simulink model "Audio_Transmission_1_"  (R2025a)
settings: Solver=VariableStepAuto  StartTime=0.0  StopTime=8  RelTol=1e-3
libraries: commanapbnd3 x6, commchan3 x3, dspsnks4 x1, dspvision x1
settings Model: Creator=sriva  LastModifiedBy=sriva

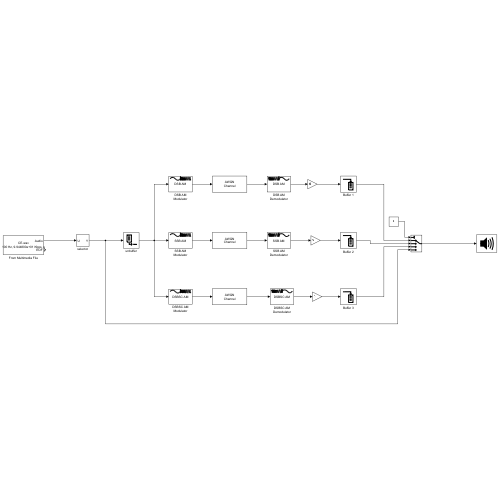
[thumbnail: Simulink's stored preview of the top-level diagram]
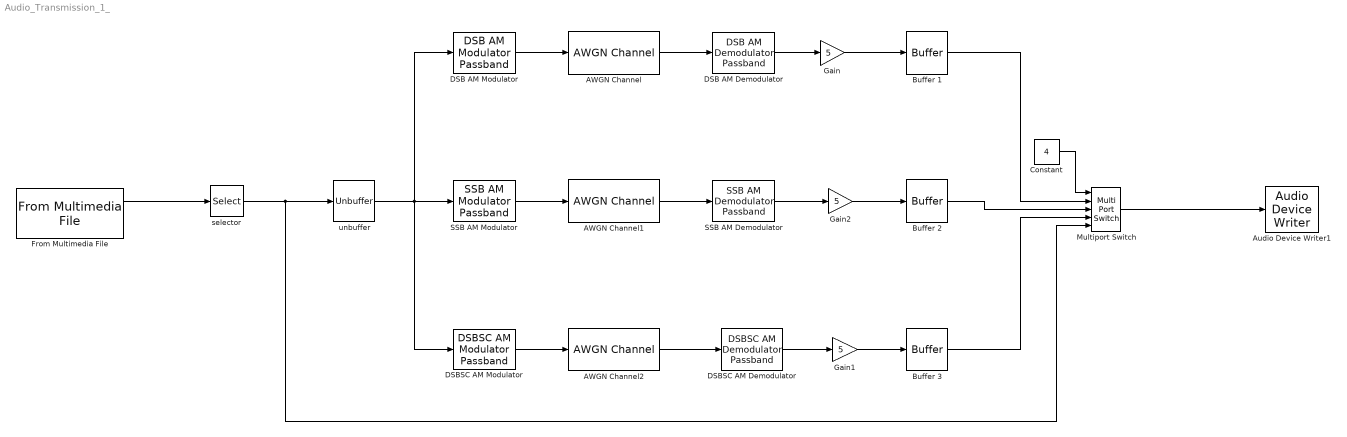
== system Audio_Transmission_1_ ==
  AWGN Channel : commchan3/AWGN Channel  LegacyMode=off  NoiseMethod="Signal to noise ratio  (SNR)"  noiseMode="Signal to noise ratio  (SNR)"  EbNo=10  EsNo=10  SNR=30  BitsPerSymbol=1  SignalPower=1  SpecifySymbolPeriod=off  SamplesPerSymbol=1  SymbolPeriod=1  VarianceSource=Parameter  Variance=1  RandomStream=Global stream  Seed=67  SimulateUsing=Code generation
  AWGN Channel1 : commchan3/AWGN Channel  LegacyMode=off  NoiseMethod="Signal to noise ratio  (SNR)"  noiseMode="Signal to noise ratio  (SNR)"  EbNo=10  EsNo=10  SNR=30  BitsPerSymbol=1  SignalPower=1  SpecifySymbolPeriod=off  SamplesPerSymbol=1  SymbolPeriod=1  VarianceSource=Parameter  Variance=1  RandomStream=Global stream  Seed=67  SimulateUsing=Code generation
  AWGN Channel2 : commchan3/AWGN Channel  LegacyMode=off  NoiseMethod="Signal to noise ratio  (SNR)"  noiseMode="Signal to noise ratio  (SNR)"  EbNo=10  EsNo=10  SNR=1000  BitsPerSymbol=1  SignalPower=1  SpecifySymbolPeriod=off  SamplesPerSymbol=1  SymbolPeriod=1  VarianceSource=Parameter  Variance=1  RandomStream=Global stream  Seed=67  SimulateUsing=Code generation
  Audio Device Writer1 : dspsnks4/Audio Device Writer  Driver=DirectSound  Device=Default  InheritSampleRate=on  SampleRate=1024  BitDepth=16-bit integer  BufferSize=4096  NumBuffers=10  DefaultOutputChannelMapping=on  OutputChannelMapping=1:2  OutputNumUnderrunSamples=off  DriverIdx=1  DeviceWarnFlag=''
  Buffer 1 : Buffer  N=1024  OutputFrames=off
  Buffer 2 : Buffer  N=1024  OutputFrames=off
  Buffer 3 : Buffer  N=1024  OutputFrames=off
  Constant : Constant  Value=4
  "DSB AM Demodulator " : commanapbnd3/DSB AM Demodulator Passband  Fc=10000  Ph=0  method=Butterworth  n=6  cf=5000  Rp=0.1  Rs=50  Offset=1
  "DSB AM Modulator " : commanapbnd3/DSB AM Modulator Passband  Fc=10000  Ph=0  Offset=1
  DSBSC AM Demodulator : commanapbnd3/DSBSC AM Demodulator Passband  Fc=10000  Ph=0  method=Butterworth  n=6  cf=5000  Rp=0.1  Rs=50
  "DSBSC AM Modulator " : commanapbnd3/DSBSC AM Modulator Passband  Fc=10000  Ph=0
  From Multimedia File : dspvision/From Multimedia File  inputFilename=C:\Users\sriva\OneDrive\Desktop\CE.wav  readRange=[1 Inf]  loop=on  numPlays=5  outputStreams=Audio only  videoDataType=single  audioDataType=double  inheritSampleTime=on  userDefinedSampleTime=1/30  noAudioOutput=off  isIntensityVideo=off  fourcc=RGB  colorVideoFormat=One multidimensional signal  outputEOF=on  dataOrg=Column-major  audioFrameSize=1024  computeAudioFrameSize=off  outSamplingMode=Sample based
      settings: LibrarySourceBlock=dspsrcs4/From Multimedia File
  Gain : Gain  Gain=5
  Gain1 : Gain  Gain=5
  Gain2 : Gain  Gain=5
  Multiport Switch : MultiPortSwitch  Inputs=4  DiagnosticForDefault=None  SaturateOnIntegerOverflow=off  InputSameDT=off
  "SSB AM Demodulator " : commanapbnd3/SSB AM Demodulator Passband  Fc=10000  Ph=0  method=Butterworth  n=6  cf=5000  Rp=0.1  Rs=50
  "SSB AM Modulator " : commanapbnd3/SSB AM Modulator Passband  Fc=10000  Ph=0  Sd=Upper  Ho=128
  selector : Selector  NumberOfDimensions=2  InputPortWidth=3  IndexOptions=Index vector (dialog),Index vector (dialog)  Indices=[1:1024],1  OutputSizes=1,1
  unbuffer : Unbuffer
  wires:
  From Multimedia File/1 -> selector/1
  selector/1 -> unbuffer/1, Multiport Switch/5
  Gain/1 -> Buffer 1/1
  "DSB AM Demodulator "/1 -> Gain/1
  unbuffer/1 -> "DSBSC AM Modulator "/1, "DSB AM Modulator "/1, "SSB AM Modulator "/1
  AWGN Channel/1 -> "DSB AM Demodulator "/1
  "SSB AM Modulator "/1 -> AWGN Channel1/1
  AWGN Channel2/1 -> DSBSC AM Demodulator/1
  Gain1/1 -> Buffer 3/1
  Gain2/1 -> Buffer 2/1
  "DSB AM Modulator "/1 -> AWGN Channel/1
  "DSBSC AM Modulator "/1 -> AWGN Channel2/1
  DSBSC AM Demodulator/1 -> Gain1/1
  "SSB AM Demodulator "/1 -> Gain2/1
  AWGN Channel1/1 -> "SSB AM Demodulator "/1
  Multiport Switch/1 -> Audio Device Writer1/1
  Buffer 1/1 -> Multiport Switch/2
  Buffer 2/1 -> Multiport Switch/3
  Buffer 3/1 -> Multiport Switch/4
  Constant/1 -> Multiport Switch/1
